simulink model "tuoyuan1"  (Simulink 6.6)
settings: Solver=ode45  StartTime=0.0  StopTime=19  RelTol=1e-3
settings Model: Creator=Administrator  LastModifiedBy=Administrator
settings OptimizationCC: InlineInvariantSignals=on
settings DebuggingCC: SignalResolutionControl=TryResolveAllWithWarning  MultiTaskDSMMsg=warning  MultiTaskCondExecSysMsg=none  StrictBusMsg=None
settings RTWCC: IncludeERTFirstTime=on

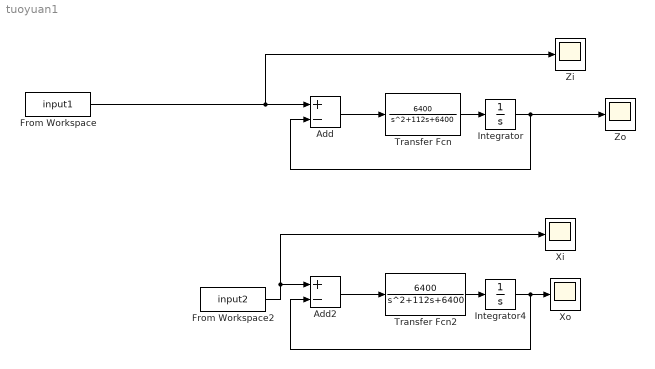
== system tuoyuan1 ==
  Add : Sum  Inputs=+-  OutScaling=2^-10
  Add2 : Sum  Inputs=+-  OutScaling=2^-10
  From Workspace : FromWorkspace  VariableName=input1  SampleTime=0
  From Workspace2 : FromWorkspace  VariableName=input2  SampleTime=0
  Integrator : Integrator
  Integrator4 : Integrator
  Transfer Fcn : TransferFcn  Numerator=[6400]  Denominator=[1 112 6400]
  Transfer Fcn2 : TransferFcn  Numerator=[6400]  Denominator=[1 112 6400]
  Xi : Scope
      settings: TimeRange=15  YMin=0  YMax=200  SaveName=Xi  DataFormat=Array
  Xo : Scope
      settings: SaveName=Xo  DataFormat=Array  MaxDataPoints=210
  Zi : Scope
      settings: TimeRange=20  YMin=0  YMax=160  SaveName=Zi  DataFormat=Array  MaxDataPoints=500
  Zo : Scope
      settings: SaveName=Zo  DataFormat=Array  MaxDataPoints=210
  wires:
  Transfer Fcn/1 -> Integrator/1
  Add/1 -> Transfer Fcn/1
  Integrator/1 -> Add/2, Zo/1
  From Workspace/1 -> Add/1, Zi/1
  Transfer Fcn2/1 -> Integrator4/1
  Add2/1 -> Transfer Fcn2/1
  From Workspace2/1 -> Add2/1, Xi/1
  Integrator4/1 -> Xo/1, Add2/2
